simulink library "xps_library"  (Simulink 7.9)
settings: Solver=ode45  SolverMode=SingleTasking  StartTime=0.0  StopTime=10.0  RelTol=1e-3
undefined symbols (not defined in the file): sys_clk, xps_library_software_register_user_data_in
libraries: xbsIndex_r4 x798, casper_library_flow_control x68, dspsigops x65, simulink x52, xps_library x35, casper_library_misc x7, xbsIndex_r3 x2
(part 4 of 10)

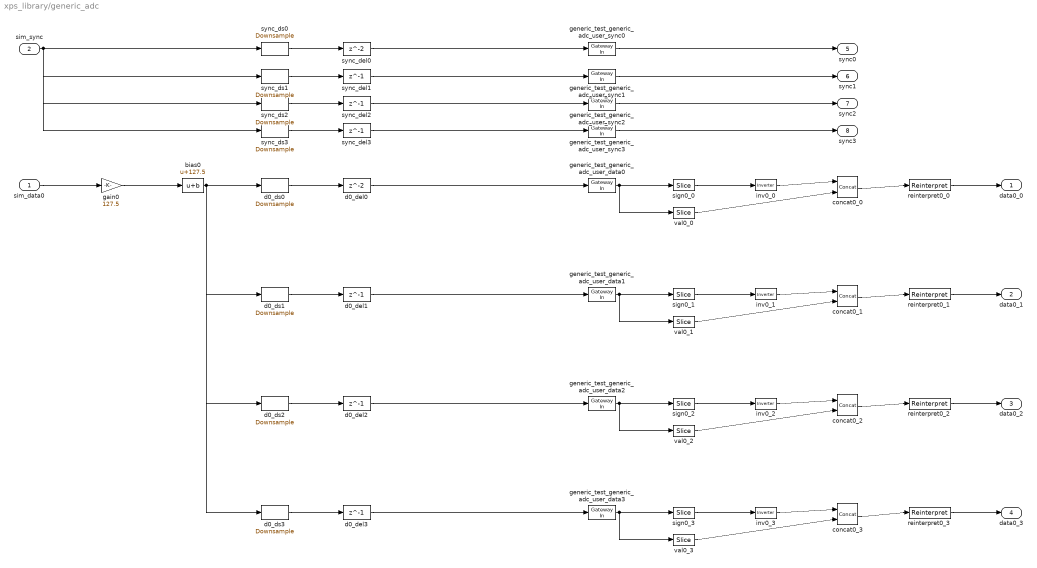
== system xps_library/generic_adc ==
  sim_data0 : Inport
  sim_sync : Inport  Port=2
  bias0 : Bias  Bias=127.5  SaturateOnIntegerOverflow=on
  concat0_{0..3} (4 alike) : xbsIndex_r4/Concat  num_inputs=2  dbl_ovrd=off  block_type=concat
  d0_del0 : Delay  InputProcessing=Inherited
  d0_del1 : Delay  DelayLength=1  InputProcessing=Inherited
  d0_del2 : Delay  DelayLength=1  InputProcessing=Inherited
  d0_del3 : Delay  DelayLength=1  InputProcessing=Inherited
  d0_ds0 : dspsigops/Downsample  N=4  phase=0  InputProcessing=Inherited (this choice will be removed - see release notes)  RateOptions=Enforce single-rate processing  smode=Allow multirate  fmode=Maintain input frame size  ic=0
  d0_ds1 : dspsigops/Downsample  N=4  phase=1  InputProcessing=Inherited (this choice will be removed - see release notes)  RateOptions=Enforce single-rate processing  smode=Allow multirate  fmode=Maintain input frame size  ic=0
  d0_ds2 : dspsigops/Downsample  N=4  phase=2  InputProcessing=Inherited (this choice will be removed - see release notes)  RateOptions=Enforce single-rate processing  smode=Allow multirate  fmode=Maintain input frame size  ic=0
  d0_ds3 : dspsigops/Downsample  N=4  phase=3  InputProcessing=Inherited (this choice will be removed - see release notes)  RateOptions=Enforce single-rate processing  smode=Allow multirate  fmode=Maintain input frame size  ic=0
  gain0 : Gain  Gain=127.5  SaturateOnIntegerOverflow=on  OutDataTypeStr=Inherit: Same as input  ParamDataTypeStr=Inherit: Same as input
  generic_test_generic_adc_user_data{0..3} (4 alike) : xbsIndex_r4/Gateway In  gui_display_data_type=Fixed-point  arith_type="Signed  (2's comp)"  n_bits=8  bin_pt=0  preci_type=Single  exp_width=8  frac_width=24  quantization="Round  (unbiased: +/- Inf)"  overflow=Saturate  period=1  dbl_ovrd=off  timing_constraint=None  locs_specified=off  LOCs={}  UseAsADC=off  ADCChannel='1'  inherit_from_input=off  hdl_port=on  block_type=gatewayin
      settings: infoedit="Gateway in block.  Converts inputs of type Simulink integer, double and fixed point to  Xilinx fixed point type.<br><br>Hardware notes:  In hardware these blocks become top level input ports."  block_version=11.4
  generic_test_generic_adc_user_sync{0..3} (4 alike) : xbsIndex_r4/Gateway In  gui_display_data_type=Fixed-point  arith_type=Boolean  n_bits=16  bin_pt=14  preci_type=Single  exp_width=8  frac_width=24  quantization="Round  (unbiased: +/- Inf)"  overflow=Saturate  period=1  dbl_ovrd=off  timing_constraint=None  locs_specified=off  LOCs={}  UseAsADC=off  ADCChannel='1'  inherit_from_input=off  hdl_port=on  block_type=gatewayin
      settings: infoedit="Gateway in block.  Converts inputs of type Simulink integer, double and fixed point to  Xilinx fixed point type.<br><br>Hardware notes:  In hardware these blocks become top level input ports."  block_version=11.4
  inv0_{0..3} (4 alike) : xbsIndex_r4/Inverter  en=off  latency=0  dbl_ovrd=off  block_type=inv
      settings: block_version=11.4
  reinterpret0_{0..3} (4 alike) : xbsIndex_r4/Reinterpret  force_arith_type=on  arith_type="Signed  (2's comp)"  force_bin_pt=on  bin_pt=7  block_type=reinterpret
      settings: infoedit="Changes signal type without altering the binary representation.   You can changed the signal between signed and unsigned, and relocate the binary point.<br><br>Hardware notes: In hardware this block costs nothing.<br><br>Example:  Suppose the input is 6 bits wide, signed, with 2 fractional bits, and the output is forced to unsigned with 0 fractional bits.  Then an input of -2.0 (1110.00 in binary 2's complement) becomes an output of 56 (111000 in binary)."
  sign0_{0..3} (4 alike) : xbsIndex_r4/Slice  nbits=1  boolean_output=off  mode=Upper Bit Location + Width  bit1=0  base1=MSB of Input  bit0=0  base0=MSB of Input  dbl_ovrd=off  block_type=slice
  sync_del0 : Delay  InputProcessing=Inherited
  sync_del1 : Delay  DelayLength=1  InputProcessing=Inherited
  sync_del2 : Delay  DelayLength=1  InputProcessing=Inherited
  sync_del3 : Delay  DelayLength=1  InputProcessing=Inherited
  sync_ds0 : dspsigops/Downsample  N=4  phase=0  InputProcessing=Inherited (this choice will be removed - see release notes)  RateOptions=Enforce single-rate processing  smode=Allow multirate  fmode=Maintain input frame size  ic=0
  sync_ds1 : dspsigops/Downsample  N=4  phase=1  InputProcessing=Inherited (this choice will be removed - see release notes)  RateOptions=Enforce single-rate processing  smode=Allow multirate  fmode=Maintain input frame size  ic=0
  sync_ds2 : dspsigops/Downsample  N=4  phase=2  InputProcessing=Inherited (this choice will be removed - see release notes)  RateOptions=Enforce single-rate processing  smode=Allow multirate  fmode=Maintain input frame size  ic=0
  sync_ds3 : dspsigops/Downsample  N=4  phase=3  InputProcessing=Inherited (this choice will be removed - see release notes)  RateOptions=Enforce single-rate processing  smode=Allow multirate  fmode=Maintain input frame size  ic=0
  val0_{0..3} (4 alike) : xbsIndex_r4/Slice  nbits=7  boolean_output=off  mode=Lower Bit Location + Width  bit1=0  base1=LSB of Input  bit0=0  base0=LSB of Input  dbl_ovrd=off  block_type=slice
  data0_0 : Outport
  data0_1 : Outport  Port=2
  data0_2 : Outport  Port=3
  data0_3 : Outport  Port=4
  sync0 : Outport  Port=5
  sync1 : Outport  Port=6
  sync2 : Outport  Port=7
  sync3 : Outport  Port=8
  wires:
  generic_test_generic_adc_user_sync3/1 -> sync3/1
  sync_del3/1 -> generic_test_generic_adc_user_sync3/1
  sync_ds3/1 -> sync_del3/1
  generic_test_generic_adc_user_sync2/1 -> sync2/1
  sync_del2/1 -> generic_test_generic_adc_user_sync2/1
  sync_ds2/1 -> sync_del2/1
  generic_test_generic_adc_user_sync1/1 -> sync1/1
  sync_del1/1 -> generic_test_generic_adc_user_sync1/1
  sync_ds1/1 -> sync_del1/1
  generic_test_generic_adc_user_sync0/1 -> sync0/1
  sync_del0/1 -> generic_test_generic_adc_user_sync0/1
  sync_ds0/1 -> sync_del0/1
  sim_sync/1 -> sync_ds3/1, sync_ds2/1, sync_ds1/1, sync_ds0/1
  reinterpret0_3/1 -> data0_3/1
  concat0_3/1 -> reinterpret0_3/1
  val0_3/1 -> concat0_3/2
  inv0_3/1 -> concat0_3/1
  sign0_3/1 -> inv0_3/1
  generic_test_generic_adc_user_data3/1 -> val0_3/1, sign0_3/1
  d0_del3/1 -> generic_test_generic_adc_user_data3/1
  d0_ds3/1 -> d0_del3/1
  reinterpret0_2/1 -> data0_2/1
  concat0_2/1 -> reinterpret0_2/1
  val0_2/1 -> concat0_2/2
  inv0_2/1 -> concat0_2/1
  sign0_2/1 -> inv0_2/1
  generic_test_generic_adc_user_data2/1 -> val0_2/1, sign0_2/1
  d0_del2/1 -> generic_test_generic_adc_user_data2/1
  d0_ds2/1 -> d0_del2/1
  reinterpret0_1/1 -> data0_1/1
  concat0_1/1 -> reinterpret0_1/1
  val0_1/1 -> concat0_1/2
  inv0_1/1 -> concat0_1/1
  sign0_1/1 -> inv0_1/1
  generic_test_generic_adc_user_data1/1 -> val0_1/1, sign0_1/1
  d0_del1/1 -> generic_test_generic_adc_user_data1/1
  d0_ds1/1 -> d0_del1/1
  reinterpret0_0/1 -> data0_0/1
  concat0_0/1 -> reinterpret0_0/1
  val0_0/1 -> concat0_0/2
  inv0_0/1 -> concat0_0/1
  sign0_0/1 -> inv0_0/1
  generic_test_generic_adc_user_data0/1 -> val0_0/1, sign0_0/1
  d0_del0/1 -> generic_test_generic_adc_user_data0/1
  d0_ds0/1 -> d0_del0/1
  bias0/1 -> d0_ds3/1, d0_ds2/1, d0_ds1/1, d0_ds0/1
  gain0/1 -> bias0/1
  sim_data0/1 -> gain0/1

== system xps_library/gpio ==
  gpio_out : Inport
  adc5g_synctest_sync_o_gateway : xbsIndex_r4/Gateway Out  inherit_from_input=off  hdl_port=on  timing_constraint=None  locs_specified=off  LOCs={}  UseAsDAC=off  DACChannel='1'  block_type=gatewayout
  convert : xbsIndex_r4/Convert  gui_display_data_type=Fixed-point  arith_type=Boolean  n_bits=1  bin_pt=0  float_type=Single  exp_bits=8  fraction_bits=24  quantization=Truncate  overflow=Wrap  en=off  latency=0  dbl_ovrd=off  pipeline=off  block_type=convert
  sim_out : Outport
  wires:
  adc5g_synctest_sync_o_gateway/1 -> sim_out/1
  convert/1 -> adc5g_synctest_sync_o_gateway/1
  gpio_out/1 -> convert/1

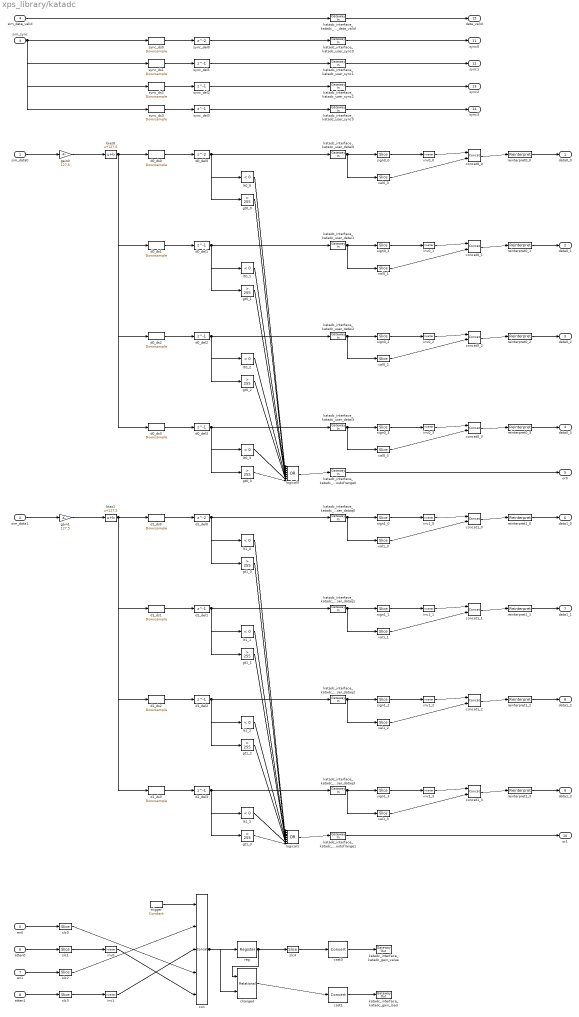
== system xps_library/katadc ==
  sim_data0 : Inport
  sim_data1 : Inport  Port=2
  sim_sync : Inport  Port=3
  sim_data_valid : Inport  Port=4
  en0 : Inport  Port=5
  atten0 : Inport  Port=6
  en1 : Inport  Port=7
  atten1 : Inport  Port=8
  bias0 : Bias  Bias=127.5  SaturateOnIntegerOverflow=on
  bias1 : Bias  Bias=127.5  SaturateOnIntegerOverflow=on
  cast0 : xbsIndex_r4/Convert  gui_display_data_type=Fixed-point  arith_type=Unsigned  n_bits=14  bin_pt=0  float_type=Single  exp_bits=8  fraction_bits=24  quantization=Truncate  overflow=Wrap  en=off  latency=0  dbl_ovrd=off  pipeline=off  block_type=convert
      settings: block_version=11.4
  cast1 : xbsIndex_r4/Convert  gui_display_data_type=Fixed-point  arith_type=Boolean  n_bits=16  bin_pt=14  float_type=Single  exp_bits=8  fraction_bits=24  quantization=Truncate  overflow=Wrap  en=off  latency=0  dbl_ovrd=off  pipeline=off  block_type=convert
      settings: block_version=11.4
  changed : xbsIndex_r4/Relational  mode=a!=b  en=off  latency=1  dbl_ovrd=off  block_type=relational
  con : xbsIndex_r4/Concat  num_inputs=5  dbl_ovrd=off  block_type=concat
  concat0_{0..3} (4 alike) : xbsIndex_r4/Concat  num_inputs=2  dbl_ovrd=off  block_type=concat
  concat1_{0..3} (4 alike) : xbsIndex_r4/Concat  num_inputs=2  dbl_ovrd=off  block_type=concat
  d0_del0 : Delay  InputProcessing=Inherited
  d0_del1 : Delay  DelayLength=1  InputProcessing=Inherited
  d0_del2 : Delay  DelayLength=1  InputProcessing=Inherited
  d0_del3 : Delay  DelayLength=1  InputProcessing=Inherited
  d0_ds0 : dspsigops/Downsample  N=4  phase=0  InputProcessing=Inherited (this choice will be removed - see release notes)  RateOptions=Enforce single-rate processing  smode=Allow multirate  fmode=Maintain input frame size  ic=0
  d0_ds1 : dspsigops/Downsample  N=4  phase=1  InputProcessing=Inherited (this choice will be removed - see release notes)  RateOptions=Enforce single-rate processing  smode=Allow multirate  fmode=Maintain input frame size  ic=0
  d0_ds2 : dspsigops/Downsample  N=4  phase=2  InputProcessing=Inherited (this choice will be removed - see release notes)  RateOptions=Enforce single-rate processing  smode=Allow multirate  fmode=Maintain input frame size  ic=0
  d0_ds3 : dspsigops/Downsample  N=4  phase=3  InputProcessing=Inherited (this choice will be removed - see release notes)  RateOptions=Enforce single-rate processing  smode=Allow multirate  fmode=Maintain input frame size  ic=0
  d1_del0 : Delay  InputProcessing=Inherited
  d1_del1 : Delay  DelayLength=1  InputProcessing=Inherited
  d1_del2 : Delay  DelayLength=1  InputProcessing=Inherited
  d1_del3 : Delay  DelayLength=1  InputProcessing=Inherited
  d1_ds0 : dspsigops/Downsample  N=4  phase=0  InputProcessing=Inherited (this choice will be removed - see release notes)  RateOptions=Enforce single-rate processing  smode=Allow multirate  fmode=Maintain input frame size  ic=0
  d1_ds1 : dspsigops/Downsample  N=4  phase=1  InputProcessing=Inherited (this choice will be removed - see release notes)  RateOptions=Enforce single-rate processing  smode=Allow multirate  fmode=Maintain input frame size  ic=0
  d1_ds2 : dspsigops/Downsample  N=4  phase=2  InputProcessing=Inherited (this choice will be removed - see release notes)  RateOptions=Enforce single-rate processing  smode=Allow multirate  fmode=Maintain input frame size  ic=0
  d1_ds3 : dspsigops/Downsample  N=4  phase=3  InputProcessing=Inherited (this choice will be removed - see release notes)  RateOptions=Enforce single-rate processing  smode=Allow multirate  fmode=Maintain input frame size  ic=0
  gain0 : Gain  Gain=127.5  SaturateOnIntegerOverflow=on  OutDataTypeStr=Inherit: Same as input  ParamDataTypeStr=Inherit: Same as input
  gain1 : Gain  Gain=127.5  SaturateOnIntegerOverflow=on  OutDataTypeStr=Inherit: Same as input  ParamDataTypeStr=Inherit: Same as input
  gt0_{0..3} (4 alike) : simulink/Logic and Bit Operations/Compare To Constant  relop=>  const=255  OutDataTypeStr=boolean  ZeroCross=off
  gt1_{0..3} (4 alike) : simulink/Logic and Bit Operations/Compare To Constant  relop=>  const=255  OutDataTypeStr=boolean  ZeroCross=off
  inv0 : xbsIndex_r4/Inverter  en=off  latency=0  dbl_ovrd=off  block_type=inv
      settings: block_version=11.4
  inv0_{0..3} (4 alike) : xbsIndex_r4/Inverter  en=off  latency=0  dbl_ovrd=off  block_type=inv
      settings: block_version=11.4
  inv1 : xbsIndex_r4/Inverter  en=off  latency=0  dbl_ovrd=off  block_type=inv
      settings: block_version=11.4
  inv1_{0..3} (4 alike) : xbsIndex_r4/Inverter  en=off  latency=0  dbl_ovrd=off  block_type=inv
      settings: block_version=11.4
  katadc_interface_katadc_gain_load : xbsIndex_r4/Gateway Out  inherit_from_input=off  hdl_port=on  timing_constraint=None  locs_specified=off  LOCs={}  UseAsDAC=off  DACChannel='1'  block_type=gatewayout
      settings: infoedit="Gateway out block.  Converts Xilinx fixed point inputs into ouputs of type Simulink integer, double, or fixed point.<br><br>Hardware notes:  In hardware these blocks become top level output ports or are discarded, depending on how they are configured."  block_version=11.4
  katadc_interface_katadc_gain_value : xbsIndex_r4/Gateway Out  inherit_from_input=off  hdl_port=on  timing_constraint=None  locs_specified=off  LOCs={}  UseAsDAC=off  DACChannel='1'  block_type=gatewayout
      settings: infoedit="Gateway out block.  Converts Xilinx fixed point inputs into ouputs of type Simulink integer, double, or fixed point.<br><br>Hardware notes:  In hardware these blocks become top level output ports or are discarded, depending on how they are configured."  block_version=11.4
  katadc_interface_katadc_user_data_valid : xbsIndex_r4/Gateway In  gui_display_data_type=Fixed-point  arith_type=Boolean  n_bits=16  bin_pt=14  preci_type=Single  exp_width=8  frac_width=24  quantization="Round  (unbiased: +/- Inf)"  overflow=Saturate  period=1  dbl_ovrd=off  timing_constraint=None  locs_specified=off  LOCs={}  UseAsADC=off  ADCChannel='1'  inherit_from_input=off  hdl_port=on  block_type=gatewayin
      settings: infoedit="Gateway in block.  Converts inputs of type Simulink integer, double and fixed point to  Xilinx fixed point type.<br><br>Hardware notes:  In hardware these blocks become top level input ports."  block_version=11.4
  katadc_interface_katadc_user_datai{0..3} (4 alike) : xbsIndex_r4/Gateway In  gui_display_data_type=Fixed-point  arith_type="Signed  (2's comp)"  n_bits=8  bin_pt=0  preci_type=Single  exp_width=8  frac_width=24  quantization="Round  (unbiased: +/- Inf)"  overflow=Saturate  period=1  dbl_ovrd=off  timing_constraint=None  locs_specified=off  LOCs={}  UseAsADC=off  ADCChannel='1'  inherit_from_input=off  hdl_port=on  block_type=gatewayin
      settings: infoedit="Gateway in block.  Converts inputs of type Simulink integer, double and fixed point to  Xilinx fixed point type.<br><br>Hardware notes:  In hardware these blocks become top level input ports."  block_version=11.4
  katadc_interface_katadc_user_dataq{0..3} (4 alike) : xbsIndex_r4/Gateway In  gui_display_data_type=Fixed-point  arith_type="Signed  (2's comp)"  n_bits=8  bin_pt=0  preci_type=Single  exp_width=8  frac_width=24  quantization="Round  (unbiased: +/- Inf)"  overflow=Saturate  period=1  dbl_ovrd=off  timing_constraint=None  locs_specified=off  LOCs={}  UseAsADC=off  ADCChannel='1'  inherit_from_input=off  hdl_port=on  block_type=gatewayin
      settings: infoedit="Gateway in block.  Converts inputs of type Simulink integer, double and fixed point to  Xilinx fixed point type.<br><br>Hardware notes:  In hardware these blocks become top level input ports."  block_version=11.4
  katadc_interface_katadc_user_outofrange0 : xbsIndex_r4/Gateway In  gui_display_data_type=Fixed-point  arith_type=Boolean  n_bits=16  bin_pt=14  preci_type=Single  exp_width=8  frac_width=24  quantization="Round  (unbiased: +/- Inf)"  overflow=Saturate  period=1  dbl_ovrd=off  timing_constraint=None  locs_specified=off  LOCs={}  UseAsADC=off  ADCChannel='1'  inherit_from_input=off  hdl_port=on  block_type=gatewayin
      settings: infoedit="Gateway in block.  Converts inputs of type Simulink integer, double and fixed point to  Xilinx fixed point type.<br><br>Hardware notes:  In hardware these blocks become top level input ports."  block_version=11.4
  katadc_interface_katadc_user_outofrange1 : xbsIndex_r4/Gateway In  gui_display_data_type=Fixed-point  arith_type=Boolean  n_bits=16  bin_pt=14  preci_type=Single  exp_width=8  frac_width=24  quantization="Round  (unbiased: +/- Inf)"  overflow=Saturate  period=1  dbl_ovrd=off  timing_constraint=None  locs_specified=off  LOCs={}  UseAsADC=off  ADCChannel='1'  inherit_from_input=off  hdl_port=on  block_type=gatewayin
      settings: infoedit="Gateway in block.  Converts inputs of type Simulink integer, double and fixed point to  Xilinx fixed point type.<br><br>Hardware notes:  In hardware these blocks become top level input ports."  block_version=11.4
  katadc_interface_katadc_user_sync{0..3} (4 alike) : xbsIndex_r4/Gateway In  gui_display_data_type=Fixed-point  arith_type=Boolean  n_bits=16  bin_pt=14  preci_type=Single  exp_width=8  frac_width=24  quantization="Round  (unbiased: +/- Inf)"  overflow=Saturate  period=1  dbl_ovrd=off  timing_constraint=None  locs_specified=off  LOCs={}  UseAsADC=off  ADCChannel='1'  inherit_from_input=off  hdl_port=on  block_type=gatewayin
      settings: infoedit="Gateway in block.  Converts inputs of type Simulink integer, double and fixed point to  Xilinx fixed point type.<br><br>Hardware notes:  In hardware these blocks become top level input ports."  block_version=11.4
  logical0 : Logic  Operator=OR  Inputs=8  AllPortsSameDT=off  OutDataTypeStr=boolean
  logical1 : Logic  Operator=OR  Inputs=8  AllPortsSameDT=off  OutDataTypeStr=boolean
  lt0_{0..3} (4 alike) : simulink/Logic and Bit Operations/Compare To Constant  relop=<  const=0  OutDataTypeStr=boolean  ZeroCross=off
  lt1_{0..3} (4 alike) : simulink/Logic and Bit Operations/Compare To Constant  relop=<  const=0  OutDataTypeStr=boolean  ZeroCross=off
  reg : xbsIndex_r4/Register  init=0  rst=off  en=off  dbl_ovrd=off  block_type=register
      settings: block_version=11.4
  reinterpret0_{0..3} (4 alike) : xbsIndex_r4/Reinterpret  force_arith_type=on  arith_type="Signed  (2's comp)"  force_bin_pt=on  bin_pt=7  block_type=reinterpret
      settings: infoedit="Changes signal type without altering the binary representation.   You can changed the signal between signed and unsigned, and relocate the binary point.<br><br>Hardware notes: In hardware this block costs nothing.<br><br>Example:  Suppose the input is 6 bits wide, signed, with 2 fractional bits, and the output is forced to unsigned with 0 fractional bits.  Then an input of -2.0 (1110.00 in binary 2's complement) becomes an output of 56 (111000 in binary)."
  reinterpret1_{0..3} (4 alike) : xbsIndex_r4/Reinterpret  force_arith_type=on  arith_type="Signed  (2's comp)"  force_bin_pt=on  bin_pt=7  block_type=reinterpret
      settings: infoedit="Changes signal type without altering the binary representation.   You can changed the signal between signed and unsigned, and relocate the binary point.<br><br>Hardware notes: In hardware this block costs nothing.<br><br>Example:  Suppose the input is 6 bits wide, signed, with 2 fractional bits, and the output is forced to unsigned with 0 fractional bits.  Then an input of -2.0 (1110.00 in binary 2's complement) becomes an output of 56 (111000 in binary)."
  sign0_{0..3} (4 alike) : xbsIndex_r4/Slice  nbits=1  boolean_output=off  mode=Upper Bit Location + Width  bit1=0  base1=MSB of Input  bit0=0  base0=MSB of Input  dbl_ovrd=off  block_type=slice
  sign1_{0..3} (4 alike) : xbsIndex_r4/Slice  nbits=1  boolean_output=off  mode=Upper Bit Location + Width  bit1=0  base1=MSB of Input  bit0=0  base0=MSB of Input  dbl_ovrd=off  block_type=slice
  slc0 : xbsIndex_r4/Slice  nbits=1  boolean_output=off  mode=Lower Bit Location + Width  bit1=0  base1=MSB of Input  bit0=0  base0=LSB of Input  dbl_ovrd=off  block_type=slice
  slc1 : xbsIndex_r4/Slice  nbits=6  boolean_output=off  mode=Lower Bit Location + Width  bit1=0  base1=MSB of Input  bit0=0  base0=LSB of Input  dbl_ovrd=off  block_type=slice
  slc2 : xbsIndex_r4/Slice  nbits=1  boolean_output=off  mode=Lower Bit Location + Width  bit1=0  base1=MSB of Input  bit0=0  base0=LSB of Input  dbl_ovrd=off  block_type=slice
  slc3 : xbsIndex_r4/Slice  nbits=6  boolean_output=off  mode=Lower Bit Location + Width  bit1=0  base1=MSB of Input  bit0=0  base0=LSB of Input  dbl_ovrd=off  block_type=slice
  slc4 : xbsIndex_r4/Slice  nbits=14  boolean_output=off  mode=Lower Bit Location + Width  bit1=0  base1=MSB of Input  bit0=0  base0=LSB of Input  dbl_ovrd=off  block_type=slice
  sync_del0 : Delay  InputProcessing=Inherited
  sync_del1 : Delay  DelayLength=1  InputProcessing=Inherited
  sync_del2 : Delay  DelayLength=1  InputProcessing=Inherited
  sync_del3 : Delay  DelayLength=1  InputProcessing=Inherited
  sync_ds0 : dspsigops/Downsample  N=4  phase=0  InputProcessing=Inherited (this choice will be removed - see release notes)  RateOptions=Enforce single-rate processing  smode=Allow multirate  fmode=Maintain input frame size  ic=0
  sync_ds1 : dspsigops/Downsample  N=4  phase=1  InputProcessing=Inherited (this choice will be removed - see release notes)  RateOptions=Enforce single-rate processing  smode=Allow multirate  fmode=Maintain input frame size  ic=0
  sync_ds2 : dspsigops/Downsample  N=4  phase=2  InputProcessing=Inherited (this choice will be removed - see release notes)  RateOptions=Enforce single-rate processing  smode=Allow multirate  fmode=Maintain input frame size  ic=0
  sync_ds3 : dspsigops/Downsample  N=4  phase=3  InputProcessing=Inherited (this choice will be removed - see release notes)  RateOptions=Enforce single-rate processing  smode=Allow multirate  fmode=Maintain input frame size  ic=0
  trigger : xbsIndex_r4/Constant  const=1  gui_display_data_type=Fixed-point  arith_type=Unsigned  n_bits=1  bin_pt=0  preci_type=Single  exp_width=8  frac_width=24  explicit_period=off  period=1  equ=P=C  opselect=C  inp2=PCIN>>17  opr=+  inp1=P  carry=CIN  dbl_ovrd=off  block_type=constant
      settings: block_version=11.4
  val0_{0..3} (4 alike) : xbsIndex_r4/Slice  nbits=7  boolean_output=off  mode=Lower Bit Location + Width  bit1=0  base1=LSB of Input  bit0=0  base0=LSB of Input  dbl_ovrd=off  block_type=slice
  val1_{0..3} (4 alike) : xbsIndex_r4/Slice  nbits=7  boolean_output=off  mode=Lower Bit Location + Width  bit1=0  base1=LSB of Input  bit0=0  base0=LSB of Input  dbl_ovrd=off  block_type=slice
  data0_0 : Outport
  data0_1 : Outport  Port=2
  data0_2 : Outport  Port=3
  data0_3 : Outport  Port=4
  or0 : Outport  Port=5
  data1_0 : Outport  Port=6
  data1_1 : Outport  Port=7
  data1_2 : Outport  Port=8
  data1_3 : Outport  Port=9
  or1 : Outport  Port=10
  sync0 : Outport  Port=11
  sync1 : Outport  Port=12
  sync2 : Outport  Port=13
  sync3 : Outport  Port=14
  data_valid : Outport  Port=15
  wires:
  cast1/1 -> katadc_interface_katadc_gain_load/1
  changed/1 -> cast1/1
  cast0/1 -> katadc_interface_katadc_gain_value/1
  slc4/1 -> cast0/1
  reg/1 -> slc4/1, changed/1
  con/1 -> changed/2, reg/1
  inv1/1 -> con/3
  slc2/1 -> con/2
  inv0/1 -> con/5
  slc0/1 -> con/4
  trigger/1 -> con/1
  slc3/1 -> inv1/1
  atten1/1 -> slc3/1
  en1/1 -> slc2/1
  slc1/1 -> inv0/1
  atten0/1 -> slc1/1
  en0/1 -> slc0/1
  katadc_interface_katadc_user_data_valid/1 -> data_valid/1
  sim_data_valid/1 -> katadc_interface_katadc_user_data_valid/1
  katadc_interface_katadc_user_sync3/1 -> sync3/1
  sync_del3/1 -> katadc_interface_katadc_user_sync3/1
  sync_ds3/1 -> sync_del3/1
  katadc_interface_katadc_user_sync2/1 -> sync2/1
  sync_del2/1 -> katadc_interface_katadc_user_sync2/1
  sync_ds2/1 -> sync_del2/1
  katadc_interface_katadc_user_sync1/1 -> sync1/1
  sync_del1/1 -> katadc_interface_katadc_user_sync1/1
  sync_ds1/1 -> sync_del1/1
  katadc_interface_katadc_user_sync0/1 -> sync0/1
  sync_del0/1 -> katadc_interface_katadc_user_sync0/1
  sync_ds0/1 -> sync_del0/1
  sim_sync/1 -> sync_ds3/1, sync_ds2/1, sync_ds1/1, sync_ds0/1
  katadc_interface_katadc_user_outofrange1/1 -> or1/1
  logical1/1 -> katadc_interface_katadc_user_outofrange1/1
  gt1_3/1 -> logical1/8
  lt1_3/1 -> logical1/7
  gt1_2/1 -> logical1/6
  lt1_2/1 -> logical1/5
  gt1_1/1 -> logical1/4
  lt1_1/1 -> logical1/3
  gt1_0/1 -> logical1/2
  lt1_0/1 -> logical1/1
  reinterpret1_3/1 -> data1_3/1
  concat1_3/1 -> reinterpret1_3/1
  val1_3/1 -> concat1_3/2
  inv1_3/1 -> concat1_3/1
  sign1_3/1 -> inv1_3/1
  katadc_interface_katadc_user_dataq3/1 -> val1_3/1, sign1_3/1
  d1_del3/1 -> gt1_3/1, lt1_3/1, katadc_interface_katadc_user_dataq3/1
  d1_ds3/1 -> d1_del3/1
  reinterpret1_2/1 -> data1_2/1
  concat1_2/1 -> reinterpret1_2/1
  val1_2/1 -> concat1_2/2
  inv1_2/1 -> concat1_2/1
  sign1_2/1 -> inv1_2/1
  katadc_interface_katadc_user_dataq2/1 -> val1_2/1, sign1_2/1
  d1_del2/1 -> gt1_2/1, lt1_2/1, katadc_interface_katadc_user_dataq2/1
  d1_ds2/1 -> d1_del2/1
  reinterpret1_1/1 -> data1_1/1
  concat1_1/1 -> reinterpret1_1/1
  val1_1/1 -> concat1_1/2
  inv1_1/1 -> concat1_1/1
  sign1_1/1 -> inv1_1/1
  katadc_interface_katadc_user_dataq1/1 -> val1_1/1, sign1_1/1
  d1_del1/1 -> gt1_1/1, lt1_1/1, katadc_interface_katadc_user_dataq1/1
  d1_ds1/1 -> d1_del1/1
  reinterpret1_0/1 -> data1_0/1
  concat1_0/1 -> reinterpret1_0/1
  val1_0/1 -> concat1_0/2
  inv1_0/1 -> concat1_0/1
  sign1_0/1 -> inv1_0/1
  katadc_interface_katadc_user_dataq0/1 -> val1_0/1, sign1_0/1
  d1_del0/1 -> gt1_0/1, lt1_0/1, katadc_interface_katadc_user_dataq0/1
  d1_ds0/1 -> d1_del0/1
  bias1/1 -> d1_ds3/1, d1_ds2/1, d1_ds1/1, d1_ds0/1
  gain1/1 -> bias1/1
  sim_data1/1 -> gain1/1
  katadc_interface_katadc_user_outofrange0/1 -> or0/1
  logical0/1 -> katadc_interface_katadc_user_outofrange0/1
  gt0_3/1 -> logical0/8
  lt0_3/1 -> logical0/7
  gt0_2/1 -> logical0/6
  lt0_2/1 -> logical0/5
  gt0_1/1 -> logical0/4
  lt0_1/1 -> logical0/3
  gt0_0/1 -> logical0/2
  lt0_0/1 -> logical0/1
  reinterpret0_3/1 -> data0_3/1
  concat0_3/1 -> reinterpret0_3/1
  val0_3/1 -> concat0_3/2
  inv0_3/1 -> concat0_3/1
  sign0_3/1 -> inv0_3/1
  katadc_interface_katadc_user_datai3/1 -> val0_3/1, sign0_3/1
  d0_del3/1 -> gt0_3/1, lt0_3/1, katadc_interface_katadc_user_datai3/1
  d0_ds3/1 -> d0_del3/1
  reinterpret0_2/1 -> data0_2/1
  concat0_2/1 -> reinterpret0_2/1
  val0_2/1 -> concat0_2/2
  inv0_2/1 -> concat0_2/1
  sign0_2/1 -> inv0_2/1
  katadc_interface_katadc_user_datai2/1 -> val0_2/1, sign0_2/1
  d0_del2/1 -> gt0_2/1, lt0_2/1, katadc_interface_katadc_user_datai2/1
  d0_ds2/1 -> d0_del2/1
  reinterpret0_1/1 -> data0_1/1
  concat0_1/1 -> reinterpret0_1/1
  val0_1/1 -> concat0_1/2
  inv0_1/1 -> concat0_1/1
  sign0_1/1 -> inv0_1/1
  katadc_interface_katadc_user_datai1/1 -> val0_1/1, sign0_1/1
  d0_del1/1 -> gt0_1/1, lt0_1/1, katadc_interface_katadc_user_datai1/1
  d0_ds1/1 -> d0_del1/1
  reinterpret0_0/1 -> data0_0/1
  concat0_0/1 -> reinterpret0_0/1
  val0_0/1 -> concat0_0/2
  inv0_0/1 -> concat0_0/1
  sign0_0/1 -> inv0_0/1
  katadc_interface_katadc_user_datai0/1 -> val0_0/1, sign0_0/1
  d0_del0/1 -> gt0_0/1, lt0_0/1, katadc_interface_katadc_user_datai0/1
  d0_ds0/1 -> d0_del0/1
  bias0/1 -> d0_ds3/1, d0_ds2/1, d0_ds1/1, d0_ds0/1
  gain0/1 -> bias0/1
  sim_data0/1 -> gain0/1

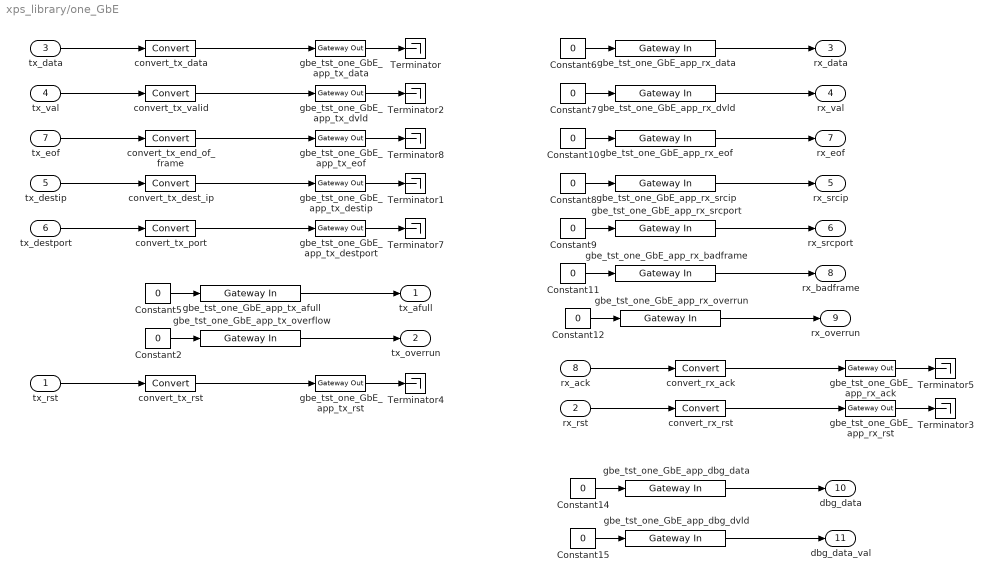
== system xps_library/one_GbE ==
  tx_rst : Inport
  rx_rst : Inport  Port=2
  tx_data : Inport  Port=3
  tx_val : Inport  Port=4
  tx_destip : Inport  Port=5
  tx_destport : Inport  Port=6
  tx_eof : Inport  Port=7
  rx_ack : Inport  Port=8
  Constant{2,5..12,14..15} (11 alike) : Constant  Value=0
  Terminator{,1..5,7..8} (8 alike) : Terminator
  convert_rx_ack : xbsIndex_r4/Convert  gui_display_data_type=Fixed-point  arith_type=Boolean  n_bits=1  bin_pt=0  float_type=Single  exp_bits=8  fraction_bits=24  quantization=Truncate  overflow=Wrap  en=off  latency=0  dbl_ovrd=off  pipeline=off  block_type=convert
      settings: xl_area=[0, 0, 0, 0, 0, 0, 0]
  convert_rx_rst : xbsIndex_r4/Convert  gui_display_data_type=Fixed-point  arith_type=Boolean  n_bits=1  bin_pt=0  float_type=Single  exp_bits=8  fraction_bits=24  quantization=Truncate  overflow=Wrap  en=off  latency=0  dbl_ovrd=off  pipeline=off  block_type=convert
      settings: xl_area=[0, 0, 0, 0, 0, 0, 0]
  convert_tx_data : xbsIndex_r4/Convert  gui_display_data_type=Fixed-point  arith_type=Unsigned  n_bits=8  bin_pt=0  float_type=Single  exp_bits=8  fraction_bits=24  quantization=Truncate  overflow=Wrap  en=off  latency=0  dbl_ovrd=off  pipeline=off  block_type=convert
      settings: xl_area=[0, 0, 0, 0, 0, 0, 0]
  convert_tx_dest_ip : xbsIndex_r4/Convert  gui_display_data_type=Fixed-point  arith_type=Unsigned  n_bits=32  bin_pt=0  float_type=Single  exp_bits=8  fraction_bits=24  quantization=Truncate  overflow=Wrap  en=off  latency=0  dbl_ovrd=off  pipeline=off  block_type=convert
      settings: xl_area=[0, 0, 0, 0, 0, 0, 0]
  convert_tx_end_of_frame : xbsIndex_r4/Convert  gui_display_data_type=Fixed-point  arith_type=Boolean  n_bits=1  bin_pt=0  float_type=Single  exp_bits=8  fraction_bits=24  quantization=Truncate  overflow=Wrap  en=off  latency=0  dbl_ovrd=off  pipeline=off  block_type=convert
      settings: xl_area=[0, 0, 0, 0, 0, 0, 0]
  convert_tx_port : xbsIndex_r4/Convert  gui_display_data_type=Fixed-point  arith_type=Unsigned  n_bits=16  bin_pt=0  float_type=Single  exp_bits=8  fraction_bits=24  quantization=Truncate  overflow=Wrap  en=off  latency=0  dbl_ovrd=off  pipeline=off  block_type=convert
      settings: xl_area=[0, 0, 0, 0, 0, 0, 0]
  convert_tx_rst : xbsIndex_r4/Convert  gui_display_data_type=Fixed-point  arith_type=Boolean  n_bits=1  bin_pt=0  float_type=Single  exp_bits=8  fraction_bits=24  quantization=Truncate  overflow=Wrap  en=off  latency=0  dbl_ovrd=off  pipeline=off  block_type=convert
      settings: xl_area=[0, 0, 0, 0, 0, 0, 0]
  convert_tx_valid : xbsIndex_r4/Convert  gui_display_data_type=Fixed-point  arith_type=Boolean  n_bits=1  bin_pt=0  float_type=Single  exp_bits=8  fraction_bits=24  quantization=Truncate  overflow=Wrap  en=off  latency=0  dbl_ovrd=off  pipeline=off  block_type=convert
      settings: xl_area=[0, 0, 0, 0, 0, 0, 0]
  gbe_tst_one_GbE_app_dbg_data : xbsIndex_r4/Gateway In  gui_display_data_type=Fixed-point  arith_type=Unsigned  n_bits=32  bin_pt=0  preci_type=Single  exp_width=8  frac_width=24  quantization=Truncate  overflow=Wrap  period=1  dbl_ovrd=off  timing_constraint=None  locs_specified=off  LOCs={}  UseAsADC=off  ADCChannel='1'  inherit_from_input=off  hdl_port=on  block_type=gatewayin
      settings: infoedit="Gateway in block.  Converts inputs of type Simulink integer, double and fixed point to  Xilinx fixed point type.<br><br>Hardware notes:  In hardware these blocks become top level input ports."  xl_area=[0, 0, 0, 0, 0, 0, 0]
  gbe_tst_one_GbE_app_dbg_dvld : xbsIndex_r4/Gateway In  gui_display_data_type=Fixed-point  arith_type=Boolean  n_bits=8  bin_pt=0  preci_type=Single  exp_width=8  frac_width=24  quantization=Truncate  overflow=Wrap  period=1  dbl_ovrd=off  timing_constraint=None  locs_specified=off  LOCs={}  UseAsADC=off  ADCChannel='1'  inherit_from_input=off  hdl_port=on  block_type=gatewayin
      settings: infoedit="Gateway in block.  Converts inputs of type Simulink integer, double and fixed point to  Xilinx fixed point type.<br><br>Hardware notes:  In hardware these blocks become top level input ports."  xl_area=[0, 0, 0, 0, 0, 0, 0]
  gbe_tst_one_GbE_app_rx_ack : xbsIndex_r4/Gateway Out  inherit_from_input=off  hdl_port=on  timing_constraint=None  locs_specified=off  LOCs={}  UseAsDAC=off  DACChannel='1'  block_type=gatewayout
      settings: infoedit="Gateway out block.  Converts Xilinx fixed point inputs into ouputs of type Simulink integer, double, or fixed point.<P><P>Hardware notes:  In hardware these blocks become top level output ports or are discarded, depending on how they are configured."  xl_area=[0, 0, 0, 0, 0, 0, 0]
  gbe_tst_one_GbE_app_rx_badframe : xbsIndex_r4/Gateway In  gui_display_data_type=Fixed-point  arith_type=Boolean  n_bits=1  bin_pt=0  preci_type=Single  exp_width=8  frac_width=24  quantization=Truncate  overflow=Wrap  period=1  dbl_ovrd=off  timing_constraint=None  locs_specified=off  LOCs={}  UseAsADC=off  ADCChannel='1'  inherit_from_input=off  hdl_port=on  block_type=gatewayin
      settings: infoedit="Gateway in block.  Converts inputs of type Simulink integer, double and fixed point to  Xilinx fixed point type.<br><br>Hardware notes:  In hardware these blocks become top level input ports."  xl_area=[0, 0, 0, 0, 0, 0, 0]
  gbe_tst_one_GbE_app_rx_data : xbsIndex_r4/Gateway In  gui_display_data_type=Fixed-point  arith_type=Unsigned  n_bits=8  bin_pt=0  preci_type=Single  exp_width=8  frac_width=24  quantization=Truncate  overflow=Wrap  period=1  dbl_ovrd=off  timing_constraint=None  locs_specified=off  LOCs={}  UseAsADC=off  ADCChannel='1'  inherit_from_input=off  hdl_port=on  block_type=gatewayin
      settings: infoedit="Gateway in block.  Converts inputs of type Simulink integer, double and fixed point to  Xilinx fixed point type.<br><br>Hardware notes:  In hardware these blocks become top level input ports."  xl_area=[0, 0, 0, 0, 0, 0, 0]
  gbe_tst_one_GbE_app_rx_dvld : xbsIndex_r4/Gateway In  gui_display_data_type=Fixed-point  arith_type=Boolean  n_bits=1  bin_pt=0  preci_type=Single  exp_width=8  frac_width=24  quantization=Truncate  overflow=Wrap  period=1  dbl_ovrd=off  timing_constraint=None  locs_specified=off  LOCs={}  UseAsADC=off  ADCChannel='1'  inherit_from_input=off  hdl_port=on  block_type=gatewayin
      settings: infoedit="Gateway in block.  Converts inputs of type Simulink integer, double and fixed point to  Xilinx fixed point type.<P><P>Hardware notes:  In hardware these blocks become top level input ports."  xl_area=[0, 0, 0, 0, 0, 0, 0]
  gbe_tst_one_GbE_app_rx_eof : xbsIndex_r4/Gateway In  gui_display_data_type=Fixed-point  arith_type=Boolean  n_bits=1  bin_pt=0  preci_type=Single  exp_width=8  frac_width=24  quantization=Truncate  overflow=Wrap  period=1  dbl_ovrd=off  timing_constraint=None  locs_specified=off  LOCs={}  UseAsADC=off  ADCChannel='1'  inherit_from_input=off  hdl_port=on  block_type=gatewayin
      settings: infoedit="Gateway in block.  Converts inputs of type Simulink integer, double and fixed point to  Xilinx fixed point type.<br><br>Hardware notes:  In hardware these blocks become top level input ports."  xl_area=[0, 0, 0, 0, 0, 0, 0]
  gbe_tst_one_GbE_app_rx_overrun : xbsIndex_r4/Gateway In  gui_display_data_type=Fixed-point  arith_type=Boolean  n_bits=1  bin_pt=0  preci_type=Single  exp_width=8  frac_width=24  quantization=Truncate  overflow=Wrap  period=1  dbl_ovrd=off  timing_constraint=None  locs_specified=off  LOCs={}  UseAsADC=off  ADCChannel='1'  inherit_from_input=off  hdl_port=on  block_type=gatewayin
      settings: infoedit="Gateway in block.  Converts inputs of type Simulink integer, double and fixed point to  Xilinx fixed point type.<br><br>Hardware notes:  In hardware these blocks become top level input ports."  xl_area=[0, 0, 0, 0, 0, 0, 0]
  gbe_tst_one_GbE_app_rx_rst : xbsIndex_r4/Gateway Out  inherit_from_input=off  hdl_port=on  timing_constraint=None  locs_specified=off  LOCs={}  UseAsDAC=off  DACChannel='1'  block_type=gatewayout
      settings: infoedit="Gateway out block.  Converts Xilinx fixed point inputs into ouputs of type Simulink integer, double, or fixed point.<P><P>Hardware notes:  In hardware these blocks become top level output ports or are discarded, depending on how they are configured."  xl_area=[0, 0, 0, 0, 0, 0, 0]
  gbe_tst_one_GbE_app_rx_srcip : xbsIndex_r4/Gateway In  gui_display_data_type=Fixed-point  arith_type=Unsigned  n_bits=32  bin_pt=0  preci_type=Single  exp_width=8  frac_width=24  quantization=Truncate  overflow=Wrap  period=1  dbl_ovrd=off  timing_constraint=None  locs_specified=off  LOCs={}  UseAsADC=off  ADCChannel='1'  inherit_from_input=off  hdl_port=on  block_type=gatewayin
      settings: infoedit="Gateway in block.  Converts inputs of type Simulink integer, double and fixed point to  Xilinx fixed point type.<br><br>Hardware notes:  In hardware these blocks become top level input ports."  xl_area=[0, 0, 0, 0, 0, 0, 0]
  gbe_tst_one_GbE_app_rx_srcport : xbsIndex_r4/Gateway In  gui_display_data_type=Fixed-point  arith_type=Unsigned  n_bits=16  bin_pt=0  preci_type=Single  exp_width=8  frac_width=24  quantization=Truncate  overflow=Wrap  period=1  dbl_ovrd=off  timing_constraint=None  locs_specified=off  LOCs={}  UseAsADC=off  ADCChannel='1'  inherit_from_input=off  hdl_port=on  block_type=gatewayin
      settings: infoedit="Gateway in block.  Converts inputs of type Simulink integer, double and fixed point to  Xilinx fixed point type.<br><br>Hardware notes:  In hardware these blocks become top level input ports."  xl_area=[0, 0, 0, 0, 0, 0, 0]
  gbe_tst_one_GbE_app_tx_afull : xbsIndex_r4/Gateway In  gui_display_data_type=Fixed-point  arith_type=Boolean  n_bits=1  bin_pt=0  preci_type=Single  exp_width=8  frac_width=24  quantization=Truncate  overflow=Wrap  period=1  dbl_ovrd=off  timing_constraint=None  locs_specified=off  LOCs={}  UseAsADC=off  ADCChannel='1'  inherit_from_input=off  hdl_port=on  block_type=gatewayin
      settings: infoedit="Gateway in block.  Converts inputs of type Simulink integer, double and fixed point to  Xilinx fixed point type.<P><P>Hardware notes:  In hardware these blocks become top level input ports."  xl_area=[0, 0, 0, 0, 0, 0, 0]
  gbe_tst_one_GbE_app_tx_data : xbsIndex_r4/Gateway Out  inherit_from_input=off  hdl_port=on  timing_constraint=None  locs_specified=off  LOCs={}  UseAsDAC=off  DACChannel='1'  block_type=gatewayout
      settings: infoedit="Gateway out block.  Converts Xilinx fixed point inputs into ouputs of type Simulink integer, double, or fixed point.<P><P>Hardware notes:  In hardware these blocks become top level output ports or are discarded, depending on how they are configured."  xl_area=[0, 0, 0, 0, 0, 0, 0]
  gbe_tst_one_GbE_app_tx_destip : xbsIndex_r4/Gateway Out  inherit_from_input=off  hdl_port=on  timing_constraint=None  locs_specified=off  LOCs={}  UseAsDAC=off  DACChannel='1'  block_type=gatewayout
      settings: infoedit="Gateway out block.  Converts Xilinx fixed point inputs into ouputs of type Simulink integer, double, or fixed point.<P><P>Hardware notes:  In hardware these blocks become top level output ports or are discarded, depending on how they are configured."  xl_area=[0, 0, 0, 0, 0, 0, 0]
  gbe_tst_one_GbE_app_tx_destport : xbsIndex_r4/Gateway Out  inherit_from_input=off  hdl_port=on  timing_constraint=None  locs_specified=off  LOCs={}  UseAsDAC=off  DACChannel='1'  block_type=gatewayout
      settings: infoedit="Gateway out block.  Converts Xilinx fixed point inputs into ouputs of type Simulink integer, double, or fixed point.<P><P>Hardware notes:  In hardware these blocks become top level output ports or are discarded, depending on how they are configured."  xl_area=[0, 0, 0, 0, 0, 0, 0]
  gbe_tst_one_GbE_app_tx_dvld : xbsIndex_r4/Gateway Out  inherit_from_input=off  hdl_port=on  timing_constraint=None  locs_specified=off  LOCs={}  UseAsDAC=off  DACChannel='1'  block_type=gatewayout
      settings: infoedit="Gateway out block.  Converts Xilinx fixed point inputs into ouputs of type Simulink integer, double, or fixed point.<P><P>Hardware notes:  In hardware these blocks become top level output ports or are discarded, depending on how they are configured."  xl_area=[0, 0, 0, 0, 0, 0, 0]
  gbe_tst_one_GbE_app_tx_eof : xbsIndex_r4/Gateway Out  inherit_from_input=off  hdl_port=on  timing_constraint=None  locs_specified=off  LOCs={}  UseAsDAC=off  DACChannel='1'  block_type=gatewayout
      settings: infoedit="Gateway out block.  Converts Xilinx fixed point inputs into ouputs of type Simulink integer, double, or fixed point.<P><P>Hardware notes:  In hardware these blocks become top level output ports or are discarded, depending on how they are configured."  xl_area=[0, 0, 0, 0, 0, 0, 0]
  gbe_tst_one_GbE_app_tx_overflow : xbsIndex_r4/Gateway In  gui_display_data_type=Fixed-point  arith_type=Boolean  n_bits=1  bin_pt=0  preci_type=Single  exp_width=8  frac_width=24  quantization=Truncate  overflow=Wrap  period=1  dbl_ovrd=off  timing_constraint=None  locs_specified=off  LOCs={}  UseAsADC=off  ADCChannel='1'  inherit_from_input=off  hdl_port=on  block_type=gatewayin
      settings: infoedit="Gateway in block.  Converts inputs of type Simulink integer, double and fixed point to  Xilinx fixed point type.<P><P>Hardware notes:  In hardware these blocks become top level input ports."  xl_area=[0, 0, 0, 0, 0, 0, 0]
  gbe_tst_one_GbE_app_tx_rst : xbsIndex_r4/Gateway Out  inherit_from_input=off  hdl_port=on  timing_constraint=None  locs_specified=off  LOCs={}  UseAsDAC=off  DACChannel='1'  block_type=gatewayout
      settings: infoedit="Gateway out block.  Converts Xilinx fixed point inputs into ouputs of type Simulink integer, double, or fixed point.<P><P>Hardware notes:  In hardware these blocks become top level output ports or are discarded, depending on how they are configured."  xl_area=[0, 0, 0, 0, 0, 0, 0]
  tx_afull : Outport
  tx_overrun : Outport  Port=2
  rx_data : Outport  Port=3
  rx_val : Outport  Port=4
  rx_srcip : Outport  Port=5
  rx_srcport : Outport  Port=6
  rx_eof : Outport  Port=7
  rx_badframe : Outport  Port=8
  rx_overrun : Outport  Port=9
  dbg_data : Outport  Port=10
  dbg_data_val : Outport  Port=11
  wires:
  gbe_tst_one_GbE_app_rx_data/1 -> rx_data/1
  tx_data/1 -> convert_tx_data/1
  convert_tx_data/1 -> gbe_tst_one_GbE_app_tx_data/1
  tx_destip/1 -> convert_tx_dest_ip/1
  convert_tx_dest_ip/1 -> gbe_tst_one_GbE_app_tx_destip/1
  tx_val/1 -> convert_tx_valid/1
  convert_tx_valid/1 -> gbe_tst_one_GbE_app_tx_dvld/1
  gbe_tst_one_GbE_app_tx_overflow/1 -> tx_overrun/1
  gbe_tst_one_GbE_app_tx_data/1 -> Terminator/1
  gbe_tst_one_GbE_app_tx_destip/1 -> Terminator1/1
  gbe_tst_one_GbE_app_tx_dvld/1 -> Terminator2/1
  Constant2/1 -> gbe_tst_one_GbE_app_tx_overflow/1
  Constant6/1 -> gbe_tst_one_GbE_app_rx_data/1
  Constant7/1 -> gbe_tst_one_GbE_app_rx_dvld/1
  gbe_tst_one_GbE_app_rx_dvld/1 -> rx_val/1
  tx_destport/1 -> convert_tx_port/1
  convert_tx_port/1 -> gbe_tst_one_GbE_app_tx_destport/1
  gbe_tst_one_GbE_app_tx_destport/1 -> Terminator7/1
  tx_eof/1 -> convert_tx_end_of_frame/1
  convert_tx_end_of_frame/1 -> gbe_tst_one_GbE_app_tx_eof/1
  gbe_tst_one_GbE_app_tx_eof/1 -> Terminator8/1
  gbe_tst_one_GbE_app_rx_srcip/1 -> rx_srcip/1
  Constant8/1 -> gbe_tst_one_GbE_app_rx_srcip/1
  Constant9/1 -> gbe_tst_one_GbE_app_rx_srcport/1
  gbe_tst_one_GbE_app_rx_srcport/1 -> rx_srcport/1
  Constant10/1 -> gbe_tst_one_GbE_app_rx_eof/1
  gbe_tst_one_GbE_app_rx_eof/1 -> rx_eof/1
  tx_rst/1 -> convert_tx_rst/1
  convert_tx_rst/1 -> gbe_tst_one_GbE_app_tx_rst/1
  gbe_tst_one_GbE_app_tx_rst/1 -> Terminator4/1
  gbe_tst_one_GbE_app_tx_afull/1 -> tx_afull/1
  Constant5/1 -> gbe_tst_one_GbE_app_tx_afull/1
  Constant11/1 -> gbe_tst_one_GbE_app_rx_badframe/1
  gbe_tst_one_GbE_app_rx_badframe/1 -> rx_badframe/1
  Constant12/1 -> gbe_tst_one_GbE_app_rx_overrun/1
  gbe_tst_one_GbE_app_rx_overrun/1 -> rx_overrun/1
  rx_rst/1 -> convert_rx_rst/1
  convert_rx_rst/1 -> gbe_tst_one_GbE_app_rx_rst/1
  gbe_tst_one_GbE_app_rx_rst/1 -> Terminator3/1
  rx_ack/1 -> convert_rx_ack/1
  convert_rx_ack/1 -> gbe_tst_one_GbE_app_rx_ack/1
  gbe_tst_one_GbE_app_rx_ack/1 -> Terminator5/1
  gbe_tst_one_GbE_app_dbg_data/1 -> dbg_data/1
  Constant14/1 -> gbe_tst_one_GbE_app_dbg_data/1
  gbe_tst_one_GbE_app_dbg_dvld/1 -> dbg_data_val/1
  Constant15/1 -> gbe_tst_one_GbE_app_dbg_dvld/1

== system xps_library/pcore ==

== system xps_library/probe ==
  probe : Inport
  Convert : xbsIndex_r3/Convert  arith_type=Boolean  n_bits=1  bin_pt=0  quantization=Truncate  overflow=Wrap  latency=0  explicit_period=off  period=1  dbl_ovrd=off  show_param=off  inserted_by_tool=off  pipeline=off
      settings: xl_area=[0, 0, 0, 0, 0, 0, 0]
  Terminator : Terminator
  xps_library_probe_TRIG0 : xbsIndex_r3/Gateway Out  output_type=Double  nbits=8  bin_pt=6  arith_type=Boolean  quantization=Truncate  overflow=Wrap  hdl_port=on  timing_constraint=None  locs_specified=off  LOCs={}  needs_fixed_name=off  show_param=off
      settings: xl_area=[0, 0, 0, 0, 0, 0, 0]
  wires:
  xps_library_probe_TRIG0/1 -> Terminator/1
  Convert/1 -> xps_library_probe_TRIG0/1
  probe/1 -> Convert/1
